simulink model "LQRFullState1"  (R2019a)
settings: Solver=VariableStepAuto  StartTime=0.0  StopTime=10.0  RelTol=1e-3
libraries: simulink x1
settings Model: Creator=florian  LastModifiedBy=florian

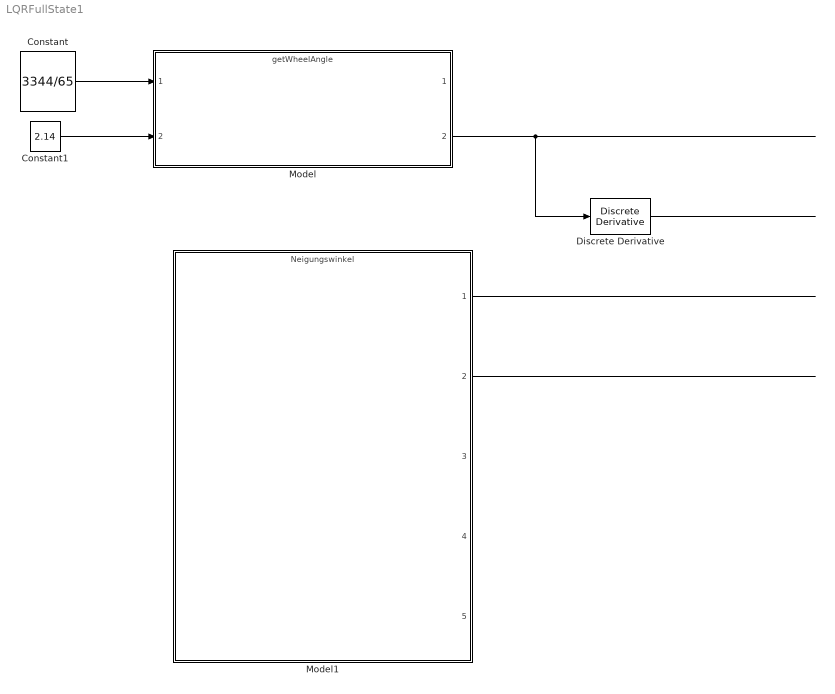
== system LQRFullState1 ==
  Constant : Constant  Value=3344/65
  Constant1 : Constant  Value=2.14
  Discrete Derivative : simulink/Discrete/Discrete Derivative  gainval=1  ICPrevScaledInput=0.0  OutMin=[]  OutMax=[]  OutDataType=fixdt(1, 16)  OutScaling=2^-10  DoSatur=off
  Model : ModelReference  ModelNameDialog=getWheelAngle.slx  SimulationMode=Normal  ModelReferenceVersion=1.8
  Model1 : ModelReference  ModelNameDialog=Neigungswinkel.slx  SimulationMode=Normal  ModelReferenceVersion=1.59
  wires:
  Model1/1 -> ?
  Model1/2 -> ?
  Constant/1 -> Model/1
  Constant1/1 -> Model/2
  Model/2 -> Discrete Derivative/1
  Discrete Derivative/1 -> ?
